simulink model "MultiLoop_mode1"  (Simulink 8.5)
settings: Solver=ode45  SolverMode=SingleTasking  StartTime=0.0  StopTime=72  FixedStep=Ts_base  MinStep=1e-6  RelTol=1e-6
PreLoadFcn:
  | Mode_1_Init
StopFcn:
  | TEplot
values from neighbouring files (symbols this model uses):
  r1_0 = 0.251/Fp_0    (= 0.00251)    [Main_GenerateTE.m]    (also in Mode_1_Init.m; Mode_3_Init.m)
  r4_0 = 9.35/Fp_0    (= 0.0935)    [Main_GenerateTE.m]    (also in Mode_1_Init.m; Mode_3_Init.m)
  Ts_base = 0.001    [Main_GenerateTE.m]    (also in Mode_1_Init.m = 0.0005; Mode_3_Init.m = 0.0005)
  Ts_save = 0.001    [Main_GenerateTE.m]    (also in Mode_1_Init.m = 0.01; Mode_3_Init.m = 0.01)
libraries: TElib x17
settings Model: Creator=ricker  LastModifiedBy=Auser  CovSFcnEnable=off
settings DataIOCC: ExternalInput=sim_input  LimitDataPoints=off  LoadExternalInput=on  LoadInitialState=on  SaveFinalState=on  SaveFormat=Structure  SaveOutput=off  SignalLogging=off  SaveTime=off  SignalLoggingName=sigsOut
settings OptimizationCC: ExpressionDepthLimit=128  InitFltsAndDblsToZero=on
settings DebuggingCC: SaveWithParameterizedLinksMsg=none  SignalResolutionControl=TryResolveAllWithWarning  MultiTaskDSMMsg=warning  MultiTaskCondExecSysMsg=none  FcnCallInpInsideContextMsg=UseLocalSettings  StateNameClashWarn=none
settings HardwareCC: TargetUnknown=on
settings GRTTargetCC: TargetFcnLib=ansi_tfl_tmw.mat

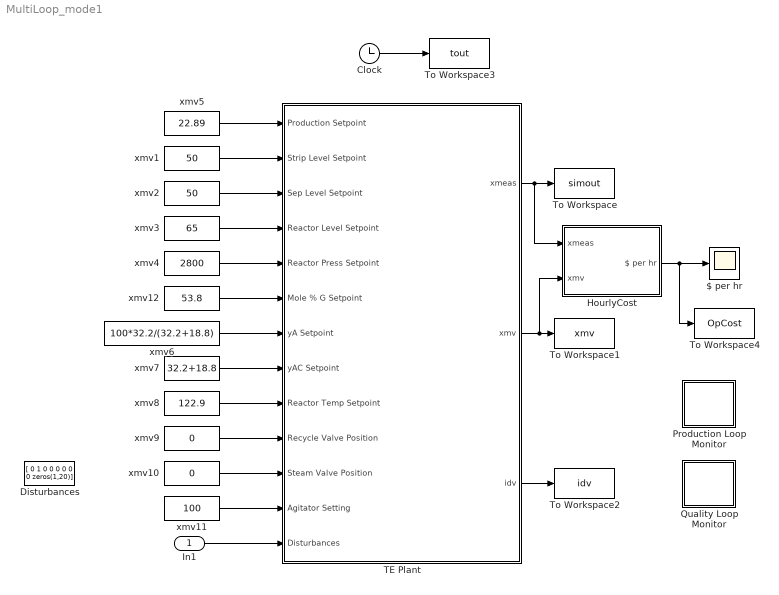
== system MultiLoop_mode1 ==
  In1 : Inport
  $ per hr : Scope
      settings: YMin=25  YMax=275  SaveName=OpCost  SampleInput=on  SampleTime=Ts_save
  Clock : Clock
  Disturbances : Constant  Value=[ 0 1 0 0 0 0 0 0 zeros(1,20)]
  HourlyCost : Subsystem
  Production Loop Monitor : Subsystem
  Quality Loop Monitor : Subsystem
  TE Plant : Subsystem
  To Workspace : ToWorkspace  VariableName=simout  SampleTime=Ts_save
  To Workspace1 : ToWorkspace  VariableName=xmv  SampleTime=Ts_save
  To Workspace2 : ToWorkspace  VariableName=idv  SampleTime=Ts_save
  To Workspace3 : ToWorkspace  VariableName=tout  SampleTime=Ts_save
  To Workspace4 : ToWorkspace  VariableName=OpCost  SampleTime=Ts_save
  xmv1 : Constant  Value=50
  xmv10 : Constant  Value=0
  xmv11 : Constant  Value=100
  xmv12 : Constant  Value=53.8
  xmv2 : Constant  Value=50
  xmv3 : Constant  Value=65
  xmv4 : Constant  Value=2800
  xmv5 : Constant  Value=22.89
  xmv6 : Constant  Value=100*32.2/(32.2+18.8)
  xmv7 : Constant  Value=32.2+18.8
  xmv8 : Constant  Value=122.9
  xmv9 : Constant  Value=0
  wires:
  TE Plant/1(xmeas) -> To Workspace/1, HourlyCost/1(xmeas)
  xmv1/1 -> TE Plant/2(Strip Level Setpoint)
  xmv2/1 -> TE Plant/3(Sep Level Setpoint)
  xmv3/1 -> TE Plant/4(Reactor Level Setpoint)
  xmv4/1 -> TE Plant/5(Reactor Press Setpoint)
  xmv8/1 -> TE Plant/9(Reactor Temp Setpoint)
  xmv6/1 -> TE Plant/7(yA Setpoint)
  xmv7/1 -> TE Plant/8(yAC Setpoint)
  TE Plant/2(xmv) -> To Workspace1/1, HourlyCost/2(xmv)
  TE Plant/3(idv) -> To Workspace2/1
  Clock/1 -> To Workspace3/1
  HourlyCost/1($ per hr) -> $ per hr/1, To Workspace4/1
  xmv9/1 -> TE Plant/10(Recycle Valve Position)
  xmv10/1 -> TE Plant/11(Steam Valve Position)
  xmv11/1 -> TE Plant/12(Agitator Setting)
  xmv12/1 -> TE Plant/6(Mole % G Setpoint)
  xmv5/1 -> TE Plant/1(Production Setpoint)
  In1/1 -> TE Plant/13(Disturbances)

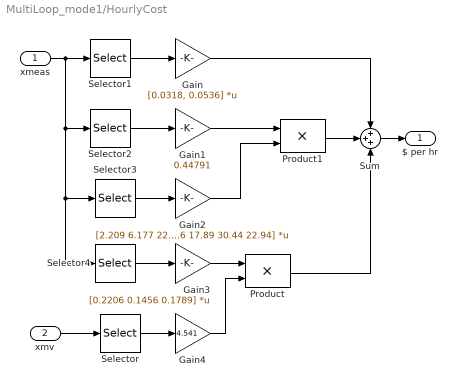
== system MultiLoop_mode1/HourlyCost ==
  xmeas : Inport  PortDimensions=41
  xmv : Inport  Port=2  PortDimensions=12
  Gain : Gain  Gain=[0.0318, 0.0536]  Multiplication=Matrix(K*u)  SaturateOnIntegerOverflow=on  OutDataTypeStr=Inherit: Same as input  ParamDataTypeStr=Inherit: Same as input
  Gain1 : Gain  Gain=0.44791  SaturateOnIntegerOverflow=on  OutDataTypeStr=Inherit: Same as input  ParamDataTypeStr=Inherit: Same as input
  Gain2 : Gain  Gain=[2.209 6.177 22.06 14.56 17.89 30.44 22.94]  Multiplication=Matrix(K*u)  SaturateOnIntegerOverflow=on  OutDataTypeStr=Inherit: Same as input  ParamDataTypeStr=Inherit: Same as input
  Gain3 : Gain  Gain=[0.2206 0.1456 0.1789]  Multiplication=Matrix(K*u)  SaturateOnIntegerOverflow=on  OutDataTypeStr=Inherit: Same as input  ParamDataTypeStr=Inherit: Same as input
  Gain4 : Gain  Gain=4.541  SaturateOnIntegerOverflow=on  OutDataTypeStr=Inherit: Same as input  ParamDataTypeStr=Inherit: Same as input
  Product : Product  SaturateOnIntegerOverflow=on  OutDataTypeStr=Inherit: Same as first input
  Product1 : Product  SaturateOnIntegerOverflow=on  OutDataTypeStr=Inherit: Same as first input
  Selector : Selector  InputPortWidth=12  Indices=8
  Selector1 : Selector  InputPortWidth=41  Indices=[19 20]
  Selector2 : Selector  InputPortWidth=41  Indices=[10]
  Selector3 : Selector  InputPortWidth=41  Indices=[29, 31:36]
  Selector4 : Selector  InputPortWidth=41  Indices=[37:39]
  Sum : Sum  Inputs=+++  SaturateOnIntegerOverflow=on
  $ per hr : Outport
  wires:
  xmv/1 -> Selector/1
  xmeas/1 -> Selector1/1, Selector2/1, Selector3/1, Selector4/1
  Selector1/1 -> Gain/1
  Selector2/1 -> Gain1/1
  Selector3/1 -> Gain2/1
  Selector4/1 -> Gain3/1
  Selector/1 -> Gain4/1
  Gain3/1 -> Product/1
  Gain4/1 -> Product/2
  Sum/1 -> $ per hr/1
  Product/1 -> Sum/3
  Gain/1 -> Sum/1
  Product1/1 -> Sum/2
  Gain1/1 -> Product1/1
  Gain2/1 -> Product1/2

== system MultiLoop_mode1/Production Loop Monitor ==
  Mux2 : Mux  Inputs=2
  Production : Scope
      settings: YMin=20  YMax=28  SaveName=Production  SampleInput=on  SampleTime=Ts_save
  wires:
  Mux2/1 -> Production/1
  [xmeas17] -> Mux2/2
  [Prodsp] -> Mux2/1

== system MultiLoop_mode1/Quality Loop Monitor ==
  Mux2 : Mux  Inputs=2
  Quality : Scope
      settings: YMin=40  YMax=60  SaveName=Quality  SampleInput=on  SampleTime=Ts_save
  wires:
  [PctGsp] -> Mux2/1
  [xmeas40] -> Mux2/2
  Mux2/1 -> Quality/1

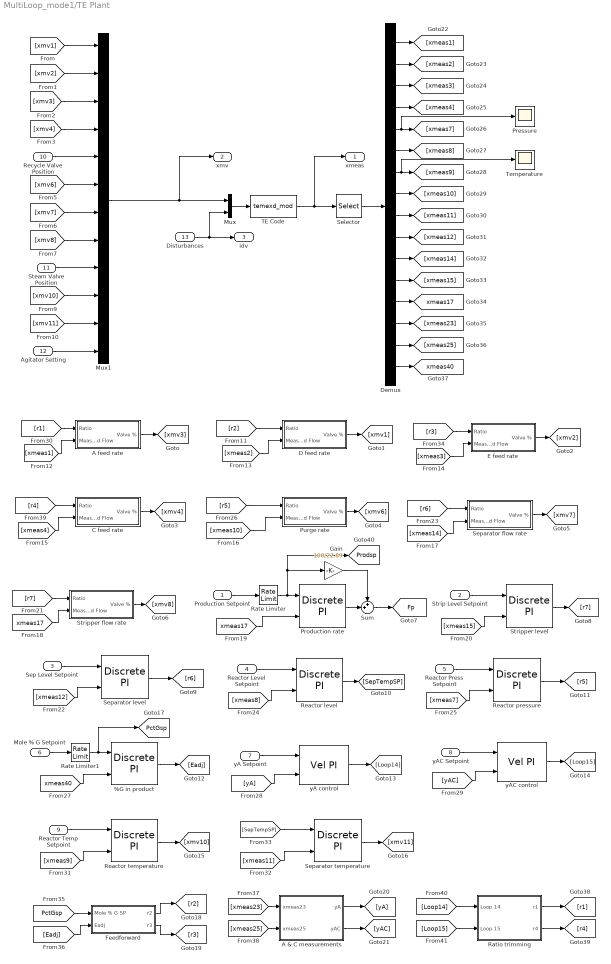
== system MultiLoop_mode1/TE Plant ==
  Production Setpoint : Inport
  Strip Level Setpoint : Inport  Port=2
  Sep Level Setpoint : Inport  Port=3
  Reactor Level Setpoint : Inport  Port=4
  Reactor Press Setpoint : Inport  Port=5
  Mole % G Setpoint : Inport  Port=6
  yA Setpoint : Inport  Port=7
  yAC Setpoint : Inport  Port=8
  Reactor Temp Setpoint : Inport  Port=9
  Recycle Valve Position : Inport  Port=10
  Steam Valve Position : Inport  Port=11
  Agitator Setting : Inport  Port=12
  Disturbances : Inport  Port=13
  %G in product : TElib/Discrete PI  Kc=-0.4  Ti=100/60  Ts=Ts_base  x0=Eadj_0  Hi=inf  Lo=-inf
  A & C measurements : Subsystem
  A feed rate : Subsystem
  C feed rate : Subsystem
  D feed rate : Subsystem
  Demux : Demux  Outputs=16
  E feed rate : Subsystem
  Feedforward : Subsystem
  Gain : Gain  Gain=100/22.89  SaturateOnIntegerOverflow=on  OutDataTypeStr=Inherit: Same as input  ParamDataTypeStr=Inherit: Same as input
  Mux : Mux  Inputs=2
  Mux1 : Mux  Inputs=12
  Pressure : Scope
      settings: YMin=2700  YMax=2900  SampleInput=on  SampleTime=Ts_save
  Production rate : TElib/Discrete PI  Kc=3.2  Ti=120/60  Ts=Ts_base  x0=0  Hi=30  Lo=-30
  Purge rate : Subsystem
  Rate Limiter : RateLimiter  RisingSlewLimit=0.3*22.95/24  FallingSlewLimit=-0.3*22.95/24
  Rate Limiter1 : RateLimiter  RisingSlewLimit=50/24  FallingSlewLimit=-50/24
  Ratio trimming : Subsystem
  Reactor level : TElib/Discrete PI  Kc=0.8  Ti=60/60  Ts=Ts_base  x0=SP17_0  Hi=120  Lo=0
  Reactor pressure : TElib/Discrete PI  Kc=-1e-4  Ti=20/60  Ts=Ts_base  x0=r5_0  Hi=100  Lo=0
  Reactor temperature : TElib/Discrete PI  Kc=-8  Ti=7.5/60  Ts=Ts_base  x0=xmv10_0  Hi=100  Lo=0
  Selector : Selector  InputPortWidth=41  Indices=[1:4, 7:12, 14, 15, 17, 23, 25, 40]
  Separator flow rate : Subsystem
  Separator level : TElib/Discrete PI  Kc=-1e-3  Ti=200/60  Ts=Ts_base  x0=r6_0  Hi=100  Lo=0
  Separator temperature : TElib/Discrete PI  Kc=-4  Ti=15/60  Ts=Ts_base  x0=xmv11_0  Hi=100  Lo=0
  Stripper flow rate : Subsystem
  Stripper level : TElib/Discrete PI  Kc=-2e-4  Ti=200/60  Ts=Ts_base  x0=r7_0  Hi=100  Lo=0
  Sum : Sum  Inputs=++|  SaturateOnIntegerOverflow=on
  TE Code : S-Function  FunctionName=temexd_mod
  Temperature : Scope
      settings: YMin=120  YMax=130  SampleInput=on  SampleTime=Ts_save
  yA control : TElib/Discrete PI/Vel PI  Kc=2e-4  Ti=1  Ts=0.1
  yAC control : TElib/Discrete PI/Vel PI  Kc=3e-4  Ti=2  Ts=0.1
  xmeas : Outport
  xmv : Outport  Port=2
  idv : Outport  Port=3
  tag scope: Fp=global, PctGsp=global, Prodsp=global, xmeas17=global, xmeas40=global
  wires:
  Mux/1 -> TE Code/1
  Disturbances/1 -> Mux/2, idv/1
  TE Code/1 -> xmeas/1, Selector/1
  [xmv1] -> Mux1/1
  [xmv2] -> Mux1/2
  [xmv3] -> Mux1/3
  [xmv4] -> Mux1/4
  Recycle Valve Position/1 -> Mux1/5
  [xmv6] -> Mux1/6
  [xmv7] -> Mux1/7
  [xmv8] -> Mux1/8
  Steam Valve Position/1 -> Mux1/9
  [xmv10] -> Mux1/10
  [xmv11] -> Mux1/11
  Agitator Setting/1 -> Mux1/12
  A feed rate/1(Valve %) -> [xmv3]
  [xmeas1] -> A feed rate/2(Measured Flow)
  D feed rate/1(Valve %) -> [xmv1]
  [xmeas2] -> D feed rate/2(Measured Flow)
  E feed rate/1(Valve %) -> [xmv2]
  [xmeas3] -> E feed rate/2(Measured Flow)
  C feed rate/1(Valve %) -> [xmv4]
  [xmeas4] -> C feed rate/2(Measured Flow)
  Purge rate/1(Valve %) -> [xmv6]
  [xmeas10] -> Purge rate/2(Measured Flow)
  Separator flow rate/1(Valve %) -> [xmv7]
  [xmeas14] -> Separator flow rate/2(Measured Flow)
  Stripper flow rate/1(Valve %) -> [xmv8]
  [xmeas17] -> Stripper flow rate/2(Measured Flow)
  [xmeas17] -> Production rate/2
  [xmeas15] -> Stripper level/2
  Strip Level Setpoint/1 -> Stripper level/1
  Stripper level/1 -> [r7]
  [r7] -> Stripper flow rate/1(Ratio)
  [xmeas12] -> Separator level/2
  Sep Level Setpoint/1 -> Separator level/1
  Separator level/1 -> [r6]
  [r6] -> Separator flow rate/1(Ratio)
  [xmeas8] -> Reactor level/2
  Reactor Level Setpoint/1 -> Reactor level/1
  Reactor level/1 -> [SepTempSP]
  [xmeas7] -> Reactor pressure/2
  Reactor Press Setpoint/1 -> Reactor pressure/1
  Reactor pressure/1 -> [r5]
  [r5] -> Purge rate/1(Ratio)
  [xmeas40] -> %G in product/2
  %G in product/1 -> [Eadj]
  [yA] -> yA control/2
  yA Setpoint/1 -> yA control/1
  yA control/1 -> [Loop14]
  [yAC] -> yAC control/2
  yAC Setpoint/1 -> yAC control/1
  yAC control/1 -> [Loop15]
  [r1] -> A feed rate/1(Ratio)
  [xmeas9] -> Reactor temperature/2
  Reactor Temp Setpoint/1 -> Reactor temperature/1
  Reactor temperature/1 -> [xmv10]
  [xmeas11] -> Separator temperature/2
  [SepTempSP] -> Separator temperature/1
  Separator temperature/1 -> [xmv11]
  [r2] -> D feed rate/1(Ratio)
  [r3] -> E feed rate/1(Ratio)
  [PctGsp] -> Feedforward/1(Mole % G SP)
  [Eadj] -> Feedforward/2(Eadj)
  Feedforward/1(r2) -> [r2]
  Feedforward/2(r3) -> [r3]
  [xmeas23] -> A & C measurements/1(xmeas23)
  [xmeas25] -> A & C measurements/2(xmeas25)
  A & C measurements/1(yA) -> [yA]
  A & C measurements/2(yAC) -> [yAC]
  Mux1/1 -> Mux/1, xmv/1
  Selector/1 -> Demux/1
  Demux/1 -> [xmeas1]
  Demux/2 -> [xmeas2]
  Demux/3 -> [xmeas3]
  Demux/4 -> [xmeas4]
  Demux/5 -> [xmeas7], Pressure/1
  Demux/6 -> [xmeas8]
  Demux/7 -> [xmeas9], Temperature/1
  Demux/8 -> [xmeas10]
  Demux/9 -> [xmeas11]
  Demux/10 -> [xmeas12]
  Demux/11 -> [xmeas14]
  Demux/12 -> [xmeas15]
  Demux/13 -> [xmeas17]
  Demux/14 -> [xmeas23]
  Demux/15 -> [xmeas25]
  Demux/16 -> [xmeas40]
  [r4] -> C feed rate/1(Ratio)
  [Loop14] -> Ratio trimming/1(Loop 14)
  [Loop15] -> Ratio trimming/2(Loop 15)
  Ratio trimming/1(r1) -> [r1]
  Ratio trimming/2(r4) -> [r4]
  Production Setpoint/1 -> Rate Limiter/1
  Rate Limiter/1 -> Production rate/1, [Prodsp], Gain/1
  Mole % G Setpoint/1 -> Rate Limiter1/1
  Rate Limiter1/1 -> %G in product/1, [PctGsp]
  Production rate/1 -> Sum/2
  Sum/1 -> [Fp]
  Gain/1 -> Sum/1

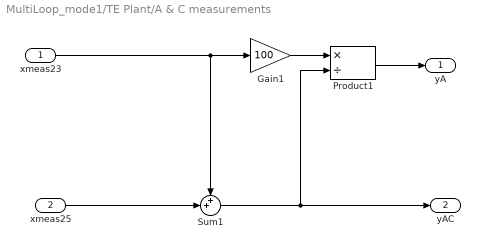
== system MultiLoop_mode1/TE Plant/A & C measurements ==
  xmeas23 : Inport
  xmeas25 : Inport  Port=2
  Gain1 : Gain  Gain=100  SaturateOnIntegerOverflow=on  OutDataTypeStr=Inherit: Same as input  ParamDataTypeStr=Inherit: Same as input
  Product1 : Product  Inputs=*/  SaturateOnIntegerOverflow=on  OutDataTypeStr=Inherit: Same as first input
  Sum1 : Sum  Inputs=++|  SaturateOnIntegerOverflow=on
  yA : Outport
  yAC : Outport  Port=2
  wires:
  Sum1/1 -> yAC/1, Product1/2
  xmeas23/1 -> Sum1/1, Gain1/1
  xmeas25/1 -> Sum1/2
  Gain1/1 -> Product1/1
  Product1/1 -> yA/1

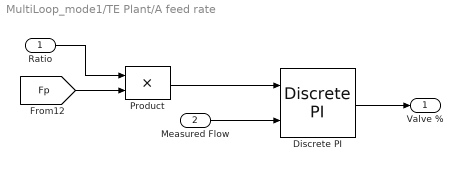
== system MultiLoop_mode1/TE Plant/A feed rate ==
  Ratio : Inport
  Measured Flow : Inport  Port=2
  Discrete PI : TElib/Discrete PI  Kc=0.01  Ti=0.001/60  Ts=Ts_base  x0=xmv3_0  Hi=100  Lo=0
  Product : Product  SaturateOnIntegerOverflow=on  OutDataTypeStr=Inherit: Same as first input
  Valve % : Outport
  wires:
  Discrete PI/1 -> Valve %/1
  Ratio/1 -> Product/1
  [Fp] -> Product/2
  Measured Flow/1 -> Discrete PI/2
  Product/1 -> Discrete PI/1

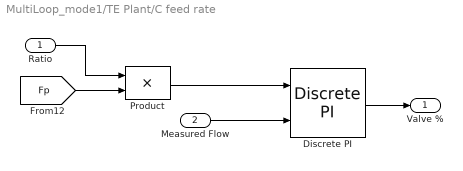
== system MultiLoop_mode1/TE Plant/C feed rate ==
  Ratio : Inport
  Measured Flow : Inport  Port=2
  Discrete PI : TElib/Discrete PI  Kc=0.003  Ti=0.001/60  Ts=Ts_base  x0=xmv4_0  Hi=100  Lo=0
  Product : Product  SaturateOnIntegerOverflow=on  OutDataTypeStr=Inherit: Same as first input
  Valve % : Outport
  wires:
  Product/1 -> Discrete PI/1
  Measured Flow/1 -> Discrete PI/2
  [Fp] -> Product/2
  Ratio/1 -> Product/1
  Discrete PI/1 -> Valve %/1

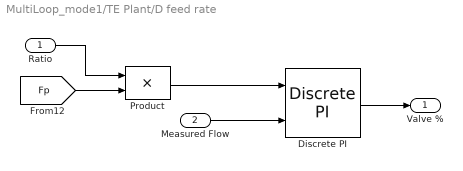
== system MultiLoop_mode1/TE Plant/D feed rate ==
  Ratio : Inport
  Measured Flow : Inport  Port=2
  Discrete PI : TElib/Discrete PI  Kc=1.6e-6  Ti=0.001/60  Ts=Ts_base  x0=xmv1_0  Hi=100  Lo=0
  Product : Product  SaturateOnIntegerOverflow=on  OutDataTypeStr=Inherit: Same as first input
  Valve % : Outport
  wires:
  Product/1 -> Discrete PI/1
  Measured Flow/1 -> Discrete PI/2
  [Fp] -> Product/2
  Ratio/1 -> Product/1
  Discrete PI/1 -> Valve %/1

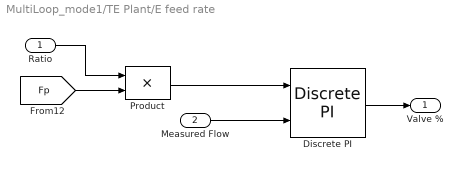
== system MultiLoop_mode1/TE Plant/E feed rate ==
  Ratio : Inport
  Measured Flow : Inport  Port=2
  Discrete PI : TElib/Discrete PI  Kc=1.8e-6  Ti=0.001/60  Ts=Ts_base  x0=xmv2_0  Hi=100  Lo=0
  Product : Product  SaturateOnIntegerOverflow=on  OutDataTypeStr=Inherit: Same as first input
  Valve % : Outport
  wires:
  Product/1 -> Discrete PI/1
  Measured Flow/1 -> Discrete PI/2
  [Fp] -> Product/2
  Ratio/1 -> Product/1
  Discrete PI/1 -> Valve %/1

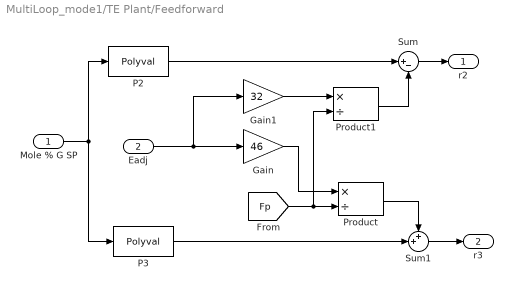
== system MultiLoop_mode1/TE Plant/Feedforward ==
  Mole % G SP : Inport
  Eadj : Inport  Port=2
  Gain : Gain  Gain=46  SaturateOnIntegerOverflow=on  OutDataTypeStr=Inherit: Same as input  ParamDataTypeStr=Inherit: Same as input
  Gain1 : Gain  Gain=32  SaturateOnIntegerOverflow=on  OutDataTypeStr=Inherit: Same as input  ParamDataTypeStr=Inherit: Same as input
  P2 : Polyval  Coefs="[1.5192e-003  5.9446e-001  2.7690e-001]"
  P3 : Polyval  Coefs="[-1.1377e-003 -8.0893e-001  9.1060e+001]"
  Product : Product  Inputs=*/  SaturateOnIntegerOverflow=on  OutDataTypeStr=Inherit: Same as first input
  Product1 : Product  Inputs=*/  SaturateOnIntegerOverflow=on  OutDataTypeStr=Inherit: Same as first input
  Sum : Sum  Inputs=|+-  SaturateOnIntegerOverflow=on
  Sum1 : Sum  Inputs=++|  SaturateOnIntegerOverflow=on
  r2 : Outport
  r3 : Outport  Port=2
  wires:
  Mole % G SP/1 -> P2/1, P3/1
  Sum/1 -> r2/1
  P2/1 -> Sum/1
  Sum1/1 -> r3/1
  P3/1 -> Sum1/2
  Product/1 -> Sum1/1
  [Fp] -> Product/2, Product1/2
  Gain/1 -> Product/1
  Eadj/1 -> Gain/1, Gain1/1
  Product1/1 -> Sum/2
  Gain1/1 -> Product1/1

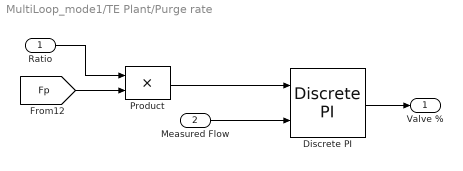
== system MultiLoop_mode1/TE Plant/Purge rate ==
  Ratio : Inport
  Measured Flow : Inport  Port=2
  Discrete PI : TElib/Discrete PI  Kc=0.01  Ti=0.001/60  Ts=Ts_base  x0=xmv6_0  Hi=100  Lo=0
  Product : Product  SaturateOnIntegerOverflow=on  OutDataTypeStr=Inherit: Same as first input
  Valve % : Outport
  wires:
  Discrete PI/1 -> Valve %/1
  Ratio/1 -> Product/1
  [Fp] -> Product/2
  Measured Flow/1 -> Discrete PI/2
  Product/1 -> Discrete PI/1

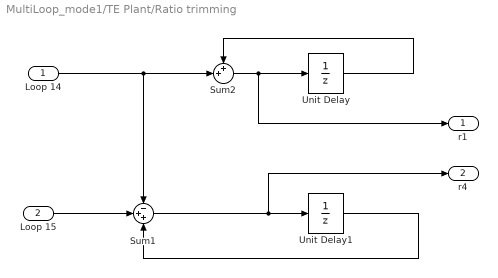
== system MultiLoop_mode1/TE Plant/Ratio trimming ==
  Loop 14 : Inport
  Loop 15 : Inport  Port=2
  Sum1 : Sum  Inputs=-++  SaturateOnIntegerOverflow=on
  Sum2 : Sum  Inputs=++|  SaturateOnIntegerOverflow=on
  Unit Delay : UnitDelay  InitialCondition=r1_0  SampleTime=0.1
  Unit Delay1 : UnitDelay  InitialCondition=r4_0  SampleTime=0.1
  r1 : Outport
  r4 : Outport  Port=2
  wires:
  Loop 15/1 -> Sum1/2
  Unit Delay/1 -> Sum2/1
  Unit Delay1/1 -> Sum1/3
  Sum2/1 -> Unit Delay/1, r1/1
  Loop 14/1 -> Sum2/2, Sum1/1
  Sum1/1 -> Unit Delay1/1, r4/1

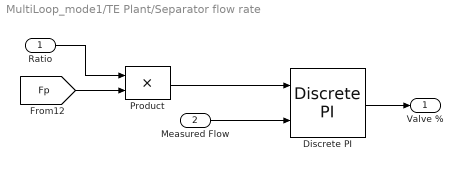
== system MultiLoop_mode1/TE Plant/Separator flow rate ==
  Ratio : Inport
  Measured Flow : Inport  Port=2
  Discrete PI : TElib/Discrete PI  Kc=4e-4  Ti=0.001/60  Ts=Ts_base  x0=xmv7_0  Hi=100  Lo=0
  Product : Product  SaturateOnIntegerOverflow=on  OutDataTypeStr=Inherit: Same as first input
  Valve % : Outport
  wires:
  Product/1 -> Discrete PI/1
  Measured Flow/1 -> Discrete PI/2
  [Fp] -> Product/2
  Ratio/1 -> Product/1
  Discrete PI/1 -> Valve %/1

== system MultiLoop_mode1/TE Plant/Stripper flow rate ==
  Ratio : Inport
  Measured Flow : Inport  Port=2
  Discrete PI : TElib/Discrete PI  Kc=4e-4  Ti=0.001/60  Ts=Ts_base  x0=xmv8_0  Hi=100  Lo=0
  Product : Product  SaturateOnIntegerOverflow=on  OutDataTypeStr=Inherit: Same as first input
  Valve % : Outport
  wires:
  Discrete PI/1 -> Valve %/1
  Ratio/1 -> Product/1
  [Fp] -> Product/2
  Measured Flow/1 -> Discrete PI/2
  Product/1 -> Discrete PI/1
